simulink model "newlinefollow"  (R2023b)
settings: Solver=FixedStepAuto  StartTime=0.0  StopTime=inf  RelTol=1e-3  EnableMultiTasking=on
libraries: vexarmcortexlib x3
settings Model: ExtModeTrigDuration=25  Creator=Monarch Robotics  LastModifiedBy=Monarch Robotics
settings OptimizationCC: EnhancedBackFolding=on  PassReuseOutputArgsAs=Individual arguments  ZeroExternalMemoryAtStartup=off  ZeroInternalMemoryAtStartup=off  MaxStackSize=64  OptimizeBlockOrder=speed  DifferentSizesBufferReuse=on  OptimizationCustomize=off  EfficientTunableParamExpr=on
settings DebuggingCC: ParameterTunabilityLossMsg=error
settings HardwareCC: ProdBitPerPointer=32  ProdBitPerSizeT=32  ProdBitPerPtrDiffT=32  ProdLargestAtomicInteger=Long  ProdLargestAtomicFloat=Double  ProdWordSize=32  ProdHWDeviceType=ARM Compatible->ARM Cortex
settings SFSimCC: MATLABDynamicMemAlloc=off
settings RTWCC: Description=Embedded Coder  SystemTargetFile=ert.tlc  HardwareBoard=ARM Cortex-based VEX Microcontroller  TLCOptions="-aInlineSetEventsForThisBaseRateFcn=TLC_FALSE -aSuppressMultiTaskScheduler=TLC_FALSE  -aRateBasedStepFcn=0"  TemplateMakefile=ert_default_tmf  Toolchain=GNU Tools for VEX ARM Cortex
settings CodeAppCC: ForceParamTrailComments=on  IgnoreCustomStorageClasses=off  OperatorAnnotations=on  SimulinkDataObjDesc=on  SFDataObjDesc=on  InsertBlockDesc=on
settings ERTTargetCC: ExtModeTransport=1  ExtModeMexFile=ext_serial_win32_comm

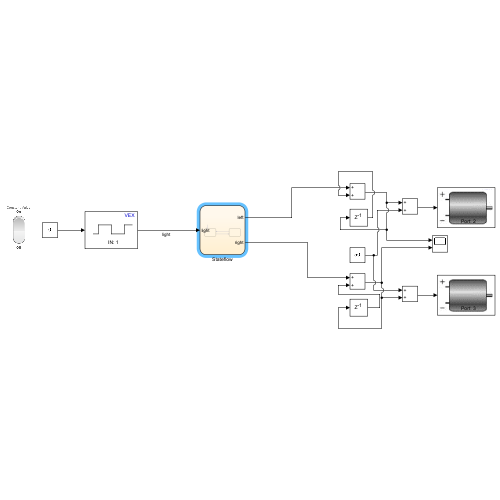
[thumbnail: Simulink's stored preview of the top-level diagram]
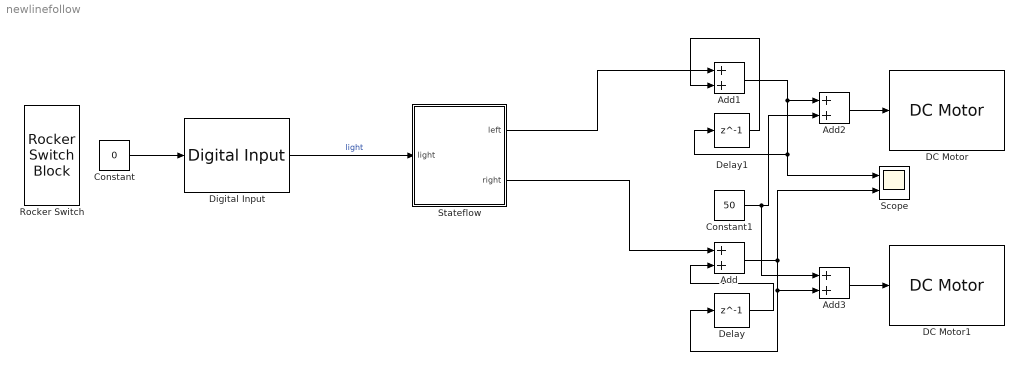
== system newlinefollow ==
  Add{,1..3} (4 alike) : Sum
  Constant : Constant  Value=0
  Constant1 : Constant  Value=50
  DC Motor : vexarmcortexlib/Actuators/DC Motor  motor=2  scaleFactor=1/13.5  SimulationOut=off
  DC Motor1 : vexarmcortexlib/Actuators/DC Motor  motor=3  scaleFactor=1/13.5  SimulationOut=off
  Delay : Delay  DelayLength=1
  Delay1 : Delay  DelayLength=1
  Digital Input : vexarmcortexlib/Sensors/Digital Input  inChan=1  SimulationIn=on  SampleTime=0.2
  Rocker Switch : RockerSwitchBlock
      settings: Values={{'Off', 'On'}, [0 1]}
  Scope : Scope  NumInputPorts=2
  Stateflow : Stateflow chart  TreatAsAtomicUnit=on
  wires:
  Add1/1 -> Add2/1, Scope/1, Delay1/1
  Delay1/1 -> Add1/2
  Delay/1 -> Add/2
  Add/1 -> Add3/2, Delay/1, Scope/2
  Stateflow/1(left) -> Add1/1
  Stateflow/2(right) -> Add/1
  Digital Input/1 -> Stateflow/1(light)  "light"
  Constant/1 -> Digital Input/1
  Add2/1 -> DC Motor/1
  Add3/1 -> DC Motor1/1
  Constant1/1 -> Add2/2, Add3/1

== stateflow chart newlinefollow/Stateflow ==
  state White
    entry:
    right=-1
    left=1
  state Black
    entry:
    right=1
    left=-1
  (default) -> White
  Black -> White : [light==1]
  White -> Black : [light==0]
  data: light input; left output; right output
